simulink model "Prob2"  (R2019b)
settings: Solver=VariableStepAuto  StartTime=0.0  StopTime=10.0  RelTol=1e-3
libraries: powerlib x10, powerlib_meascontrol x1
settings Model: Creator=bhanu prasad  LastModifiedBy=bhanu prasad

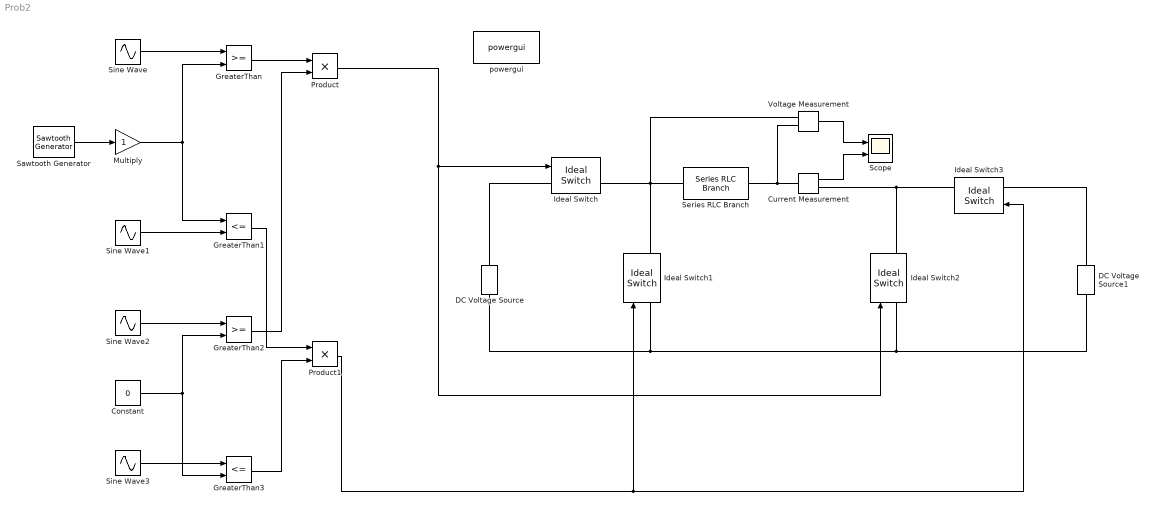
== system Prob2 ==
  Constant : Constant  Value=0
  Current Measurement : powerlib/Measurements/Current Measurement  PhasorSimulation=off  OutputType=Complex  PSBequivalent=0
      settings: SourceProductName=Simscape Electrical
  DC Voltage Source : powerlib/Electrical Sources/DC Voltage Source  Amplitude=100  Measurements=None
      settings: SourceProductName=Simscape Electrical
  DC Voltage Source1 : powerlib/Electrical Sources/DC Voltage Source  Amplitude=100  Measurements=None
      settings: SourceProductName=Simscape Electrical
  GreaterThan : RelationalOperator  OutDataTypeStr=boolean  RndMeth=Simplest
  GreaterThan1 : RelationalOperator  Operator=<=  OutDataTypeStr=boolean  RndMeth=Simplest
  GreaterThan2 : RelationalOperator  OutDataTypeStr=boolean  RndMeth=Simplest
  GreaterThan3 : RelationalOperator  Operator=<=  OutDataTypeStr=boolean  RndMeth=Simplest
  Ideal Switch{,1..3} (4 alike) : powerlib/Power Electronics/Ideal Switch  Ron=0.001  Lon=0  IC=0  Rs=1e5  Cs=inf  Measurements=on
      settings: SourceProductName=Simscape Electrical
  Multiply : Gain
  Product : Product
  Product1 : Product
  Sawtooth Generator : powerlib_meascontrol/Pulse & Signal Generators/Sawtooth Generator  Freq=1050  Phase=180  Ts=0
      settings: SourceProductName=Simscape Electrical
  Scope : Scope  NumInputPorts=2
  Series RLC Branch : powerlib/Elements/Series RLC Branch  LConnTagsString=__new0  RConnTagsString=__new0  BranchType=R  Resistance=1  Inductance=1e-3  SetiL0=off  InitialCurrent=0  Capacitance=1e-6  Setx0=off  InitialVoltage=0  Measurements=None
      settings: SourceProductName=Simscape Electrical
  Sine Wave{,1..3} (4 alike) : Sin  Frequency=2*pi/0.02  SampleTime=0
  Voltage Measurement : powerlib/Measurements/Voltage Measurement  PhasorSimulation=off  OutputType=Complex  PSBequivalent=0
      settings: SourceProductName=Simscape Electrical
  powergui : powerlib/powergui  Priority=1  SimulationMode=Continuous  SampleTime=50e-6  frequency=60  Iterations=50  frequencyindice=0  Pbase=100e6  ErrMax=1e-4  UnitsV=kV  UnitsW=MW  buscounter=0  FunctionMessages=off  echomessages=off  EnableUseOfTLC=off  CurrentSourceSwitches=off  DisableSnubberDevices=off  DisableRonSwitches=off  DisableVfSwitches=off  DisplayEquations=off  AutomaticDiscreteSolvers=off  SolverType=Tustin/Backward Euler (TBE)  Interpol=off  ExternalGateDelay=off  methode=off  Ts=100  x0status=blocks  SPID=on  SwTol=0  HookPort=off  NonlinearTolerance=1e-4  nMaxIteration=100  ContinueOnMaxIteration=off  RestoreLinks=warning  ResistiveCurrentMeasurement=off  Frange=[0:2:500]  Ylog=off  Xlog=on  ShowGrid=off  save=off  variable=ZData  structure=0  ZoomFFT=off  StartTime=0.0  cycles=1  DisplayStyle=1  fundamental=60  FreqAxis=off  MaxFrequency=1000  frequencyindicesteady=1  RmsSteady=1  display=off
      settings: SourceProductName=Simscape Electrical
  wires:
  Voltage Measurement/1 -> Scope/1
  Current Measurement/1 -> Scope/2
  Sawtooth Generator/1 -> Multiply/1
  Sine Wave/1 -> GreaterThan/1
  Multiply/1 -> GreaterThan1/1, GreaterThan/2
  Sine Wave1/1 -> GreaterThan1/2
  Sine Wave2/1 -> GreaterThan2/1
  Sine Wave3/1 -> GreaterThan3/1
  Constant/1 -> GreaterThan3/2, GreaterThan2/2
  GreaterThan/1 -> Product/1
  GreaterThan2/1 -> Product/2
  GreaterThan1/1 -> Product1/1
  GreaterThan3/1 -> Product1/2
  Product/1 -> Ideal Switch/1, Ideal Switch2/1
  Product1/1 -> Ideal Switch1/1, Ideal Switch3/1
  connections:
  Current Measurement/LConn1 -- Voltage Measurement/LConn2 -- Series RLC Branch/RConn1
  Ideal Switch/RConn1 -- Series RLC Branch/LConn1 -- Voltage Measurement/LConn1 -- Ideal Switch1/RConn1
  Current Measurement/RConn1 -- Ideal Switch2/RConn1 -- Ideal Switch3/RConn1
  DC Voltage Source/RConn1 -- Ideal Switch/LConn1
  DC Voltage Source1/RConn1 -- Ideal Switch3/LConn1
  DC Voltage Source/LConn1 -- DC Voltage Source1/LConn1 -- Ideal Switch2/LConn1 -- Ideal Switch1/LConn1
